simulink model "scratch"  (R2020a)
settings: Solver=VariableStepAuto  StartTime=0.0  StopTime=10.0  RelTol=1e-3
undefined symbols (not defined in the file or in its folder): opt, srad
libraries: simulink x3, powerlib x1
settings Model: Creator=shrad  LastModifiedBy=shrad
settings SolverCC: AlgebraicLoopSolver=LineSearch

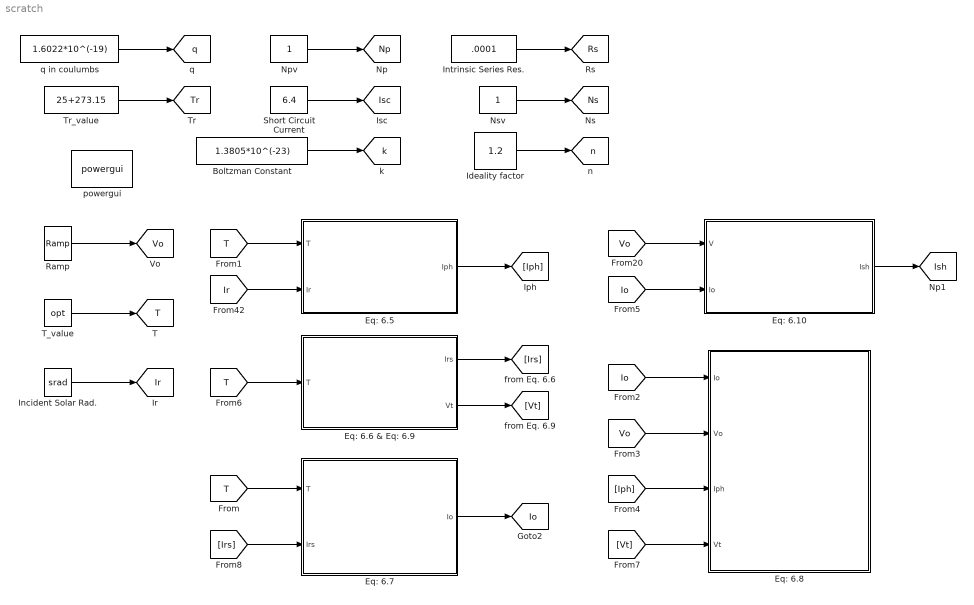
== system scratch ==
  Boltzman Constant : Constant  Value=1.3805*10^(-23)
  Eq: 6.10 : Subsystem
  Eq: 6.5 : Subsystem
  Eq: 6.6 & Eq: 6.9 : Subsystem
  Eq: 6.7 : Subsystem
  Eq: 6.8 : Subsystem
  Ideality factor : Constant  Value=1.2
  Incident Solar Rad. : Constant  Value=srad
  Intrinsic Series Res. : Constant  Value=.0001
  Npv : Constant
  Nsv : Constant
  Ramp : simulink/Sources/Ramp  slope=3  start=0  InitialOutput=0
  Short Circuit Current : Constant  Value=6.4
  T_value : Constant  Value=opt
  Tr_value : Constant  Value=25+273.15
  powergui : powerlib/powergui  Priority=1  SimulationMode=Discrete  SampleTime=1e-6  frequency=60  Iterations=50  frequencyindice=0  Pbase=100e6  ErrMax=1e-4  UnitsV=kV  UnitsW=MW  buscounter=0  FunctionMessages=off  echomessages=off  EnableUseOfTLC=off  CurrentSourceSwitches=off  DisableSnubberDevices=off  DisableRonSwitches=off  DisableVfSwitches=off  DisplayEquations=off  AutomaticDiscreteSolvers=off  SolverType=Tustin  Interpol=off  ExternalGateDelay=off  methode=off  Ts=0  x0status=blocks  SPID=off  SwTol=0  HookPort=off  NonlinearTolerance=1e-4  nMaxIteration=100  ContinueOnMaxIteration=off  RestoreLinks=warning  ResistiveCurrentMeasurement=off  Frange=[0:2:500]  Ylog=off  Xlog=on  ShowGrid=off  save=off  variable=ZData  structure=0  ZoomFFT=off  StartTime=0.0  cycles=1  DisplayStyle=1  fundamental=60  FreqAxis=off  MaxFrequency=1000  frequencyindicesteady=1  RmsSteady=1  display=off
  q in coulumbs : Constant  Value=1.6022*10^(-19)
  tag scope: Io=global, Ir=global, Isc=global, Ish=global, Np=global, Ns=global, Rs=global, T=global, Tr=global, Vo=global, k=global, n=global, q=global
  wires:
  T_value/1 -> [T]
  Incident Solar Rad./1 -> [Ir]
  Ramp/1 -> [Vo]
  Eq: 6.5/1(Iph) -> [Iph]
  [T] -> Eq: 6.5/1(T)
  [Ir] -> Eq: 6.5/2(Ir)
  Short Circuit Current/1 -> [Isc]
  Tr_value/1 -> [Tr]
  Eq: 6.6 & Eq: 6.9/1(Irs) -> [Irs]
  [T] -> Eq: 6.6 & Eq: 6.9/1(T)
  Eq: 6.6 & Eq: 6.9/2(Vt) -> [Vt]
  [Irs] -> Eq: 6.7/2(Irs)
  Eq: 6.7/1(Io) -> [Io]
  [T] -> Eq: 6.7/1(T)
  Nsv/1 -> [Ns]
  Boltzman Constant/1 -> [k]
  Ideality factor/1 -> [n]
  q in coulumbs/1 -> [q]
  Eq: 6.10/1(Ish) -> [Ish]
  [Io] -> Eq: 6.10/2(Io)
  [Vo] -> Eq: 6.10/1(V)
  Npv/1 -> [Np]
  Intrinsic Series Res./1 -> [Rs]
  [Vo] -> Eq: 6.8/2(Vo)
  [Iph] -> Eq: 6.8/3(Iph)
  [Vt] -> Eq: 6.8/4(Vt)
  [Io] -> Eq: 6.8/1(Io)

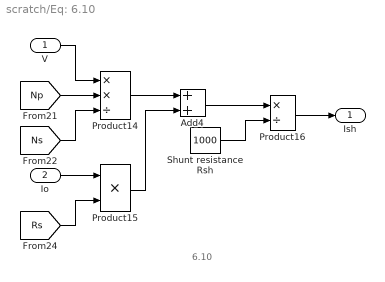
== system scratch/Eq: 6.10 ==
  note: 6.10
  V : Inport
  Io : Inport  Port=2
  Add4 : Sum
  Product14 : Product  Inputs=**/
  Product15 : Product
  Product16 : Product  Inputs=*/
  Shunt resistance Rsh : Constant  Value=1000
  Ish : Outport
  wires:
  Add4/1 -> Product16/1
  Io/1 -> Product15/1
  Product16/1 -> Ish/1
  Shunt resistance Rsh/1 -> Product16/2
  [Np] -> Product14/2
  Product14/1 -> Add4/1
  [Ns] -> Product14/3
  Product15/1 -> Add4/2
  V/1 -> Product14/1
  [Rs] -> Product15/2

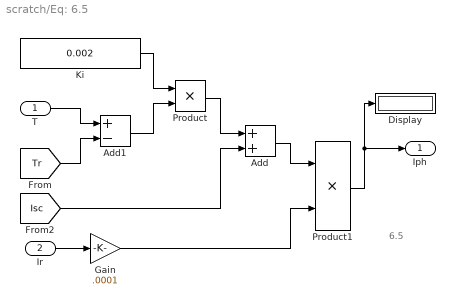
== system scratch/Eq: 6.5 ==
  note: 6.5
  T : Inport
  Ir : Inport  Port=2
  Add : Sum
  Add1 : Sum  Inputs=+-
  Display : Display
  Gain : Gain  Gain=.0001
  Ki : Constant  Value=0.002
  Product : Product
  Product1 : Product
  Iph : Outport
  wires:
  Product/1 -> Add/1
  Add1/1 -> Product/2
  T/1 -> Add1/1
  Ki/1 -> Product/1
  [Tr] -> Add1/2
  Product1/1 -> Iph/1, Display/1
  [Isc] -> Add/2
  Ir/1 -> Gain/1
  Add/1 -> Product1/1
  Gain/1 -> Product1/2

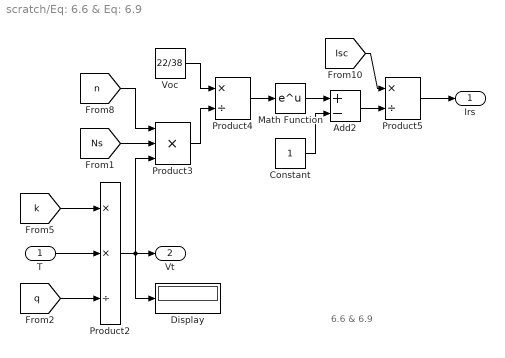
== system scratch/Eq: 6.6 & Eq: 6.9 ==
  note: 6.6 & 6.9
  T : Inport
  Add2 : Sum  Inputs=+-
  Constant : Constant
  Display : Display
  Math Function : Math  SaturateOnIntegerOverflow=on
  Product2 : Product  Inputs=**/
  Product3 : Product  Inputs=3
  Product4 : Product  Inputs=*/
  Product5 : Product  Inputs=*/
  Voc : Constant  Value=22/38
  Irs : Outport
  Vt : Outport  Port=2
  wires:
  Product4/1 -> Math Function/1
  [k] -> Product2/1
  [q] -> Product2/3
  [Isc] -> Product5/1
  Add2/1 -> Product5/2
  Constant/1 -> Add2/2
  [n] -> Product3/1
  Product3/1 -> Product4/2
  Voc/1 -> Product4/1
  Math Function/1 -> Add2/1
  Product2/1 -> Display/1, Product3/3, Vt/1
  Product5/1 -> Irs/1
  T/1 -> Product2/2
  [Ns] -> Product3/2

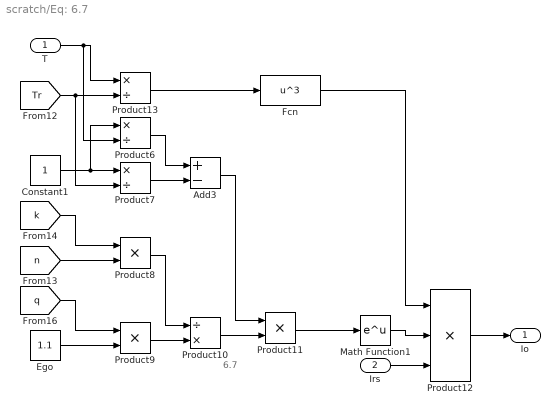
== system scratch/Eq: 6.7 ==
  note: 6.7
  T : Inport
  Irs : Inport  Port=2
  Add3 : Sum  Inputs=+-
  Constant1 : Constant
  Ego : Constant  Value=1.1
  Fcn : Fcn  Expr=u^3
  Math Function1 : Math  SaturateOnIntegerOverflow=on
  Product10 : Product  Inputs=/*
  Product11 : Product  Inputs=**
  Product12 : Product  Inputs=***
  Product13 : Product  Inputs=*/
  Product6 : Product  Inputs=*/
  Product7 : Product  Inputs=*/
  Product8 : Product  Inputs=**
  Product9 : Product  Inputs=**
  Io : Outport
  wires:
  Product12/1 -> Io/1
  [q] -> Product9/1
  Product6/1 -> Add3/1
  Product10/1 -> Product11/2
  Product11/1 -> Math Function1/1
  Product8/1 -> Product10/1
  Ego/1 -> Product9/2
  Product13/1 -> Fcn/1
  Product9/1 -> Product10/2
  Fcn/1 -> Product12/1
  [n] -> Product8/2
  Product7/1 -> Add3/2
  [k] -> Product8/1
  Add3/1 -> Product11/1
  Math Function1/1 -> Product12/2
  Irs/1 -> Product12/3
  [Tr] -> Product13/2, Product7/2
  T/1 -> Product6/2, Product13/1
  Constant1/1 -> Product6/1, Product7/1

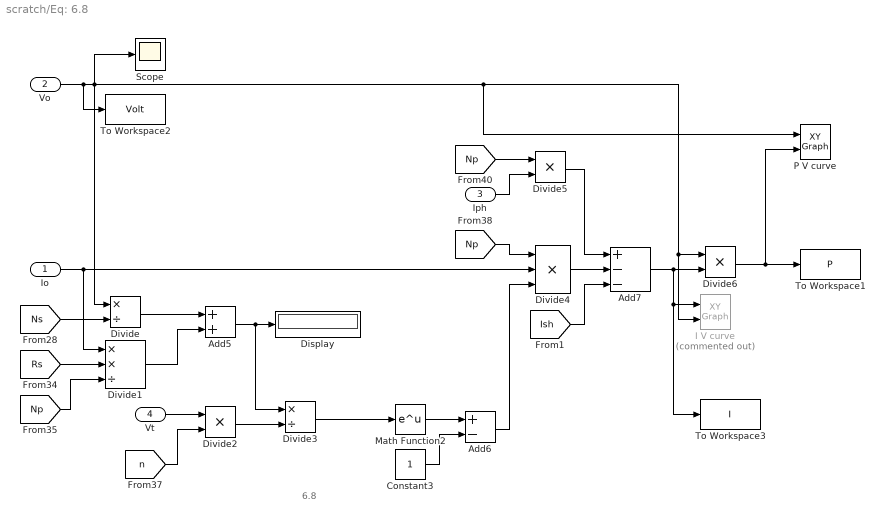
== system scratch/Eq: 6.8 ==
  note: 6.8
  Io : Inport
  Vo : Inport  Port=2
  Iph : Inport  Port=3
  Vt : Inport  Port=4
  Add5 : Sum
  Add6 : Sum  Inputs=+-
  Add7 : Sum  Inputs=+--
  Constant3 : Constant
  Display : Display
  Divide : Product  Inputs=*/
  Divide1 : Product  Inputs=**/
  Divide2 : Product
  Divide3 : Product  Inputs=*/
  Divide4 : Product  Inputs=3
  Divide5 : Product
  Divide6 : Product
  I V curve : simulink/Sinks/XY Graph  Commented=on  xmin=-1  xmax=22  ymin=-1  ymax=10  st=-1
  Math Function2 : Math  SaturateOnIntegerOverflow=on
  P V curve : simulink/Sinks/XY Graph  xmin=-1  xmax=1  ymin=-1  ymax=1  st=-1
  Scope : Scope
  To Workspace1 : ToWorkspace  VariableName=P  SaveFormat=Timeseries  SampleTime=-1
  To Workspace2 : ToWorkspace  VariableName=Volt  SaveFormat=Timeseries  SampleTime=-1
  To Workspace3 : ToWorkspace  VariableName=I  SaveFormat=Timeseries  SampleTime=-1
  wires:
  [Ns] -> Divide/2
  [n] -> Divide2/2
  [Np] -> Divide5/1
  Divide2/1 -> Divide3/2
  Divide5/1 -> Add7/1
  Divide1/1 -> Add5/2
  [Np] -> Divide4/1
  Math Function2/1 -> Add6/1
  [Ish] -> Add7/3
  [Rs] -> Divide1/2
  Iph/1 -> Divide5/2
  [Np] -> Divide1/3
  Add6/1 -> Divide4/3
  Constant3/1 -> Add6/2
  Vt/1 -> Divide2/1
  Divide3/1 -> Math Function2/1
  Divide4/1 -> Add7/2
  Divide/1 -> Add5/1
  Add7/1 -> I V curve/1, To Workspace3/1, Divide6/2
  Divide6/1 -> P V curve/2, To Workspace1/1
  Vo/1 -> Scope/1, I V curve/2, Divide6/1, P V curve/1, Divide/1, To Workspace2/1
  Add5/1 -> Display/1, Divide3/1
  Io/1 -> Divide1/1, Divide4/2
